simulink model "suspend_kamotu_kato"  (R2020b)
settings: Solver=ode45  StartTime=0.0  StopTime=100
undefined symbols (not defined in the file or in its folder): traj
settings Model: Creator=iketa  LastModifiedBy=kt012
settings DebuggingCC: ArithmeticOperatorsInVariantConditions=warning
settings SFSimCC: CustomCodeUndefinedFunction=UseInterfaceOnly

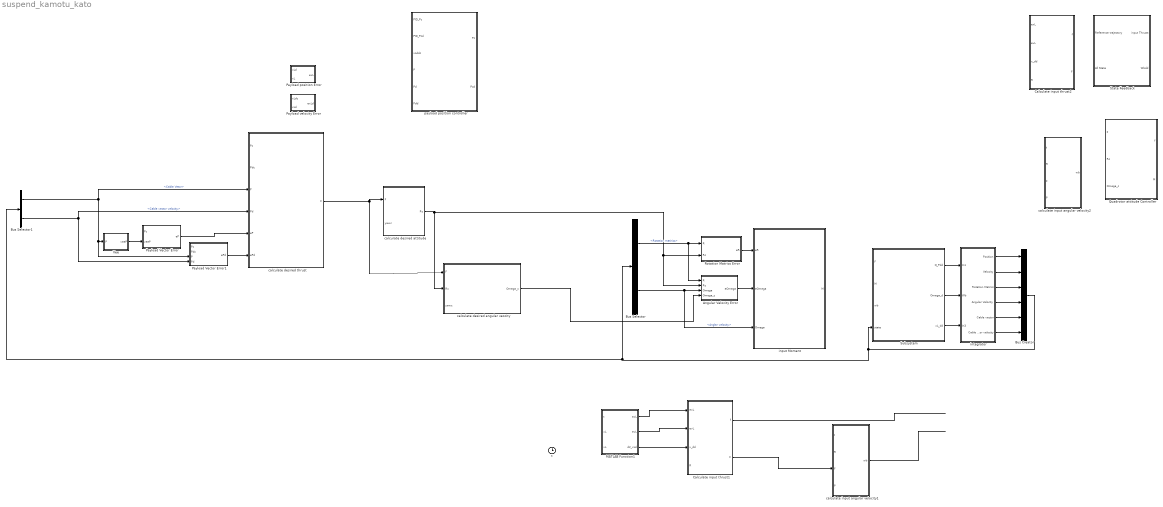
== system suspend_kamotu_kato ==
  Angular Velocity Error : MATLAB Function  TreatAsAtomicUnit=on
  Bus Creator : BusCreator  Inputs=6
  Bus Selector : BusSelector  OutputSignals=Rotation matirics,Anglar velosity
  Bus Selector1 : BusSelector  OutputSignals=Cable Vetor,Cable vector velocity
  Calculate input thrust1 : MATLAB Function
  Calculate input thrust2 : MATLAB Function
  MATLAB Function1 : MATLAB Function  TreatAsAtomicUnit=on
  Payload Vector Error : MATLAB Function  TreatAsAtomicUnit=on
  Payload Vector Error1 : MATLAB Function  TreatAsAtomicUnit=on
  Payload position Error : MATLAB Function  TreatAsAtomicUnit=on
  Payload velocity Error : MATLAB Function  TreatAsAtomicUnit=on
  Quadrotor attitude Controller : MATLAB Function  TreatAsAtomicUnit=on
  Rotation Matrics Error : MATLAB Function  TreatAsAtomicUnit=on
  State Feedback : Subsystem
  Subsystem : Subsystem
  Vee : MATLAB Function  TreatAsAtomicUnit=on
  calculate desired angular veocity : MATLAB Function  TreatAsAtomicUnit=on
  calculate desired thrust : MATLAB Function  TreatAsAtomicUnit=on
  calculate input angular velocity1 : MATLAB Function  TreatAsAtomicUnit=on
  calculate input angular velocity2 : MATLAB Function  TreatAsAtomicUnit=on
  calcurate desired attitude : MATLAB Function  TreatAsAtomicUnit=on
  input Moment : MATLAB Function  TreatAsAtomicUnit=on
  integrator : Subsystem
  payload position controller : MATLAB Function  TreatAsAtomicUnit=on
  t : Clock
  wires:
  Subsystem/1(Q_Pdd) -> integrator/1(In1)
  Subsystem/2(Omega_d) -> integrator/2(Wb)
  Subsystem/3(xL_dd) -> integrator/3(In3)
  ? -> Calculate input thrust1/4(R), calculate input angular velocity1/2(R)
  ? -> MATLAB Function1/3(vL)
  ? -> MATLAB Function1/2(xL), calculate input angular velocity1/4(P)
  calculate input angular velocity1/1(wb) -> ?
  Calculate input thrust1/1(f) -> ?
  Calculate input thrust1/2(F) -> calculate input angular velocity1/3(F)
  MATLAB Function1/3(d2_xLd) -> Calculate input thrust1/3(x_dd)
  MATLAB Function1/2(evL) -> Calculate input thrust1/2(evL)
  ? -> calculate input angular velocity1/1(t)
  MATLAB Function1/1(exL) -> Calculate input thrust1/1(exL)
  integrator/1(Position) -> Bus Creator/1
  integrator/6(Cable vector velocity) -> Bus Creator/6
  integrator/2(Velocity) -> Bus Creator/2
  integrator/3(Rotation Matrics) -> Bus Creator/3
  integrator/5(Cable vector) -> Bus Creator/5
  Bus Creator/1 -> Bus Selector1/1, Bus Selector/1, Subsystem/4(state)
  Angular Velocity Error/1(eOmega) -> input Moment/2(eOmega)
  Rotation Matrics Error/1(eR) -> input Moment/1(eR)
  integrator/4(Angular Velocity) -> Bus Creator/4
  Bus Selector/2 -> input Moment/3(Omega), Angular Velocity Error/3(Omega)  "<Anglar velosity>"
  Bus Selector/1 -> Angular Velocity Error/1(R), Rotation Matrics Error/1(R)  "<Rotation matirics>"
  Vee/1(veeP) -> Payload Vector Error/2(veeP)
  Payload Vector Error/1(eP) -> calculate desired thrust/5(eP)
  Payload Vector Error1/1(ePd) -> calculate desired thrust/6(ePd)
  calculate desired thrust/1(F) -> calcurate desired attitude/1(F), calculate desired angular veocity/1(F)
  calcurate desired attitude/1(Rc) -> Angular Velocity Error/2(Rc), Rotation Matrics Error/2(Rc), calculate desired angular veocity/2(Rc)
  Bus Selector1/1 -> calculate desired thrust/3(P), Payload Vector Error1/3(P), Vee/1(P)  "<Cable Vetor>"
  Bus Selector1/2 -> Payload Vector Error1/4(Pd), calculate desired thrust/4(Pd)  "<Cable vector velocity>"
  calculate desired angular veocity/1(Omega_c) -> Angular Velocity Error/4(Omega_c)

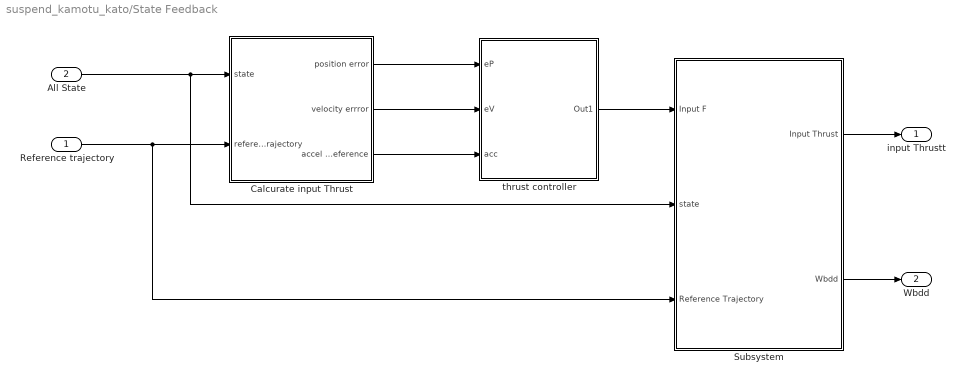
== system suspend_kamotu_kato/State Feedback ==
  Reference trajectory : Inport
  All State : Inport  Port=2
  Calcurate input Thrust : Subsystem
  Subsystem : Subsystem
  thrust controller : Subsystem
  input Thrustt : Outport
  "Wbdd " : Outport  Port=2  VectorParamsAs1DForOutWhenUnconnected=off
  wires:
  thrust controller/1(Out1) -> Subsystem/1(Input F)
  Calcurate input Thrust/3(accel reference) -> thrust controller/3(acc)
  Calcurate input Thrust/2(velocity errror) -> thrust controller/2(eV)
  Calcurate input Thrust/1(position error) -> thrust controller/1(eP)
  Subsystem/1(Input Thrust) -> input Thrustt/1
  Subsystem/2("Wbdd ") -> "Wbdd "/1
  Reference trajectory/1 -> Subsystem/3(Reference Trajectory), Calcurate input Thrust/2(reference trajectory)
  All State/1 -> Subsystem/2(state), Calcurate input Thrust/1(state)

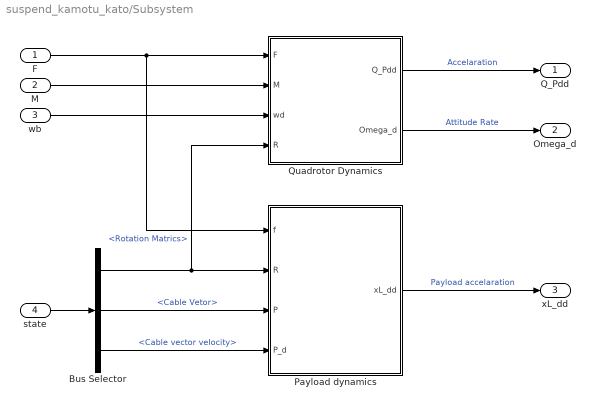
== system suspend_kamotu_kato/Subsystem ==
  F : Inport
  M : Inport  Port=2
  wb : Inport  Port=3
  state : Inport  Port=4
  Bus Selector : BusSelector  OutputSignals=Rotation Matrics,Cable Vetor,Cable vector velocity
  Payload dynamics : MATLAB Function  TreatAsAtomicUnit=on
  Quadrotor Dynamics : MATLAB Function  TreatAsAtomicUnit=on
  Q_Pdd : Outport
  Omega_d : Outport  Port=2
  xL_dd : Outport  Port=3
  wires:
  Payload dynamics/1(xL_dd) -> xL_dd/1  "Payload accelaration"
  Bus Selector/2 -> Payload dynamics/3(P)  "<Cable Vetor>"
  F/1 -> Payload dynamics/1(f), Quadrotor Dynamics/1(F)
  Quadrotor Dynamics/2(Omega_d) -> Omega_d/1  "Attitude Rate"
  Quadrotor Dynamics/1(Q_Pdd) -> Q_Pdd/1  "Accelaration"
  wb/1 -> Quadrotor Dynamics/3(wd)
  state/1 -> Bus Selector/1
  Bus Selector/1 -> Quadrotor Dynamics/4(R), Payload dynamics/2(R)  "<Rotation Matrics>"
  Bus Selector/3 -> Payload dynamics/4(P_d)  "<Cable vector velocity>"
  M/1 -> Quadrotor Dynamics/2(M)

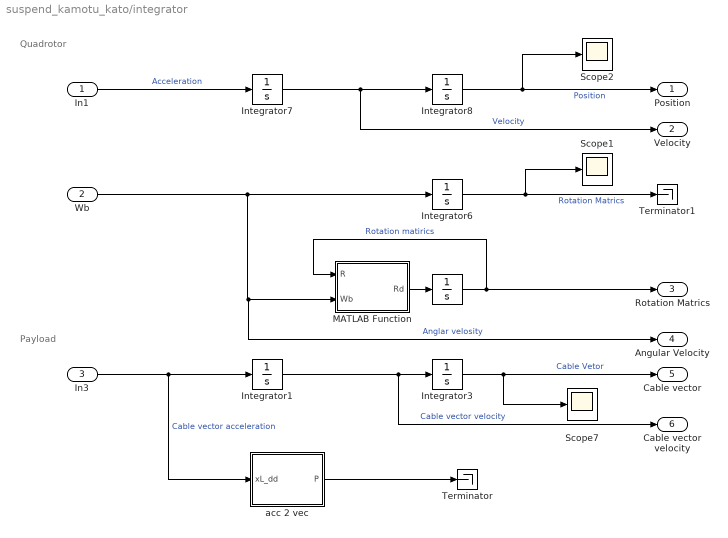
== system suspend_kamotu_kato/integrator ==
  note: Quadrotor
  note: Payload
  In1 : Inport
  Wb : Inport  Port=2
  In3 : Inport  Port=3
  " " : Integrator  InitialCondition=[1 0 0; 0 1 0; 0 0 1];  ContinuousStateAttributes="\"\""
  Integrator{1,3,6..8} (5 alike) : Integrator  InitialCondition=[0;0;0]
  MATLAB Function : MATLAB Function  TreatAsAtomicUnit=on
  Scope1 : Scope
  Scope2 : Scope
  Scope7 : Scope
  Terminator : Terminator
  Terminator1 : Terminator
  acc 2 vec : MATLAB Function  TreatAsAtomicUnit=on
  Position : Outport
  Velocity : Outport  Port=2
  Rotation Matrics : Outport  Port=3
  Angular Velocity : Outport  Port=4
  Cable vector : Outport  Port=5
  Cable vector velocity : Outport  Port=6
  wires:
  In3/1 -> Integrator1/1, acc 2 vec/1(xL_dd)  "Cable vector acceleration"
  Integrator1/1 -> Cable vector velocity/1, Integrator3/1  "Cable vector velocity"
  acc 2 vec/1(P) -> Terminator/1
  Integrator3/1 -> Cable vector/1, Scope7/1  "Cable Vetor"
  Integrator6/1 -> Terminator1/1, Scope1/1  "Rotation Matrics"
  Integrator7/1 -> Velocity/1, Integrator8/1  "Velocity"
  Integrator8/1 -> Position/1, Scope2/1  "Position"
  In1/1 -> Integrator7/1  "Acceleration"
  MATLAB Function/1(Rd) -> " "/1
  Wb/1 -> Angular Velocity/1, MATLAB Function/2(Wb), Integrator6/1  "Anglar velosity"
  " "/1 -> Rotation Matrics/1, MATLAB Function/1(R)  "Rotation matirics"

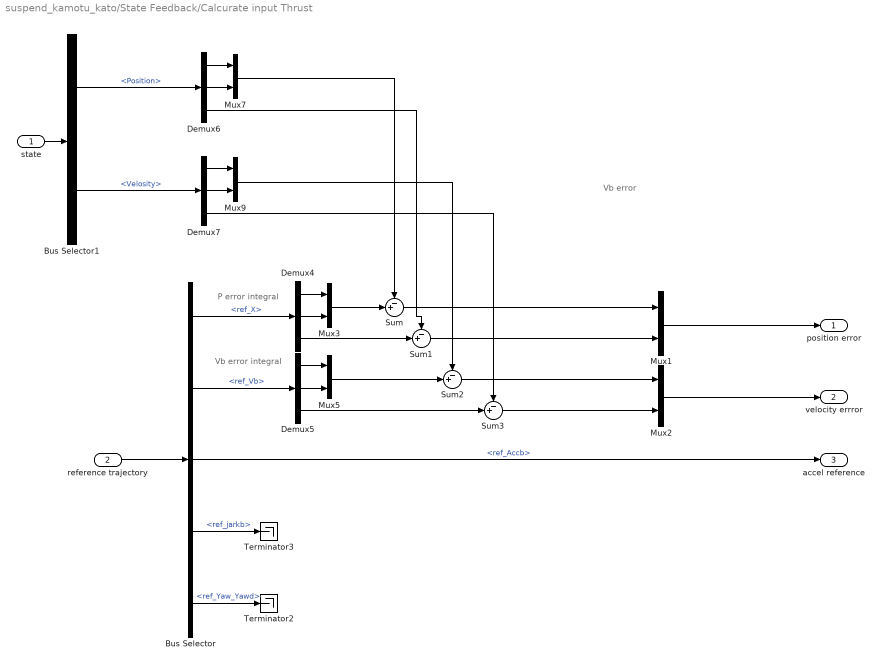
== system suspend_kamotu_kato/State Feedback/Calcurate input Thrust ==
  note: Vb error integral
  note: Vb error
  note: P error integral
  state : Inport
  reference trajectory : Inport  Port=2
  Bus Selector : BusSelector  OutputSignals=ref_X,ref_Vb,ref_Accb,ref_jarkb,ref_Yaw_Yawd
  Bus Selector1 : BusSelector  OutputSignals=Position,Velosity
  Demux{4..7} (4 alike) : Demux  Outputs=3
  Mux{1..3,5,7,9} (6 alike) : Mux  Inputs=2
  Sum{,1..3} (4 alike) : Sum  Inputs=-+|
  Terminator2 : Terminator
  Terminator3 : Terminator
  position error : Outport
  velocity errror : Outport  Port=2
  accel reference : Outport  Port=3
  wires:
  Mux3/1 -> Sum/2
  Demux5/1 -> Mux5/1
  Demux6/3 -> Sum1/1
  Demux7/2 -> Mux9/2
  Bus Selector/2 -> Demux5/1  "<ref_Vb>"
  Demux7/1 -> Mux9/1
  Sum/1 -> Mux1/1
  Demux5/2 -> Mux5/2
  Demux4/2 -> Mux3/2
  Bus Selector1/2 -> Demux7/1  "<Velosity>"
  Sum1/1 -> Mux1/2
  Mux9/1 -> Sum2/1
  Mux7/1 -> Sum/1
  Mux1/1 -> position error/1
  Demux7/3 -> Sum3/1
  Demux6/1 -> Mux7/1
  Bus Selector1/1 -> Demux6/1  "<Position>"
  Sum2/1 -> Mux2/1
  Demux4/3 -> Sum1/2
  state/1 -> Bus Selector1/1
  Bus Selector/3 -> accel reference/1  "<ref_Accb>"
  Demux4/1 -> Mux3/1
  Mux2/1 -> velocity errror/1
  Bus Selector/4 -> Terminator3/1  "<ref_jarkb>"
  Sum3/1 -> Mux2/2
  Bus Selector/5 -> Terminator2/1  "<ref_Yaw_Yawd>"
  Mux5/1 -> Sum2/2
  reference trajectory/1 -> Bus Selector/1
  Bus Selector/1 -> Demux4/1  "<ref_X>"
  Demux5/3 -> Sum3/2
  Demux6/2 -> Mux7/2

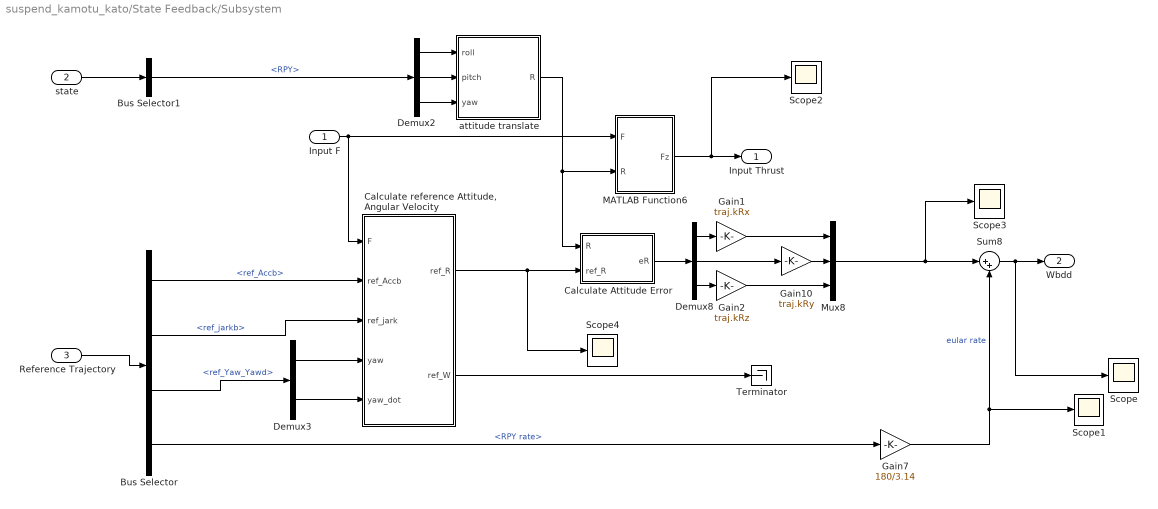
== system suspend_kamotu_kato/State Feedback/Subsystem ==
  Input F : Inport
  state : Inport  Port=2
  Reference Trajectory : Inport  Port=3
  Bus Selector : BusSelector  OutputSignals=ref_Accb,ref_jarkb,ref_Yaw_Yawd,RPY rate
  Bus Selector1 : BusSelector  OutputSignals=RPY
  Calculate Attitude Error : MATLAB Function  TreatAsAtomicUnit=on
  "Calculate reference Attitude, Angular Velocity" : MATLAB Function  TreatAsAtomicUnit=on
  Demux2 : Demux  Outputs=3
  Demux3 : Demux  Outputs=2
  Demux8 : Demux  Outputs=3
  Gain1 : Gain  Gain=traj.kRx
  Gain10 : Gain  Gain=traj.kRy
  Gain2 : Gain  Gain=traj.kRz
  Gain7 : Gain  Gain=180/3.14
  MATLAB Function6 : MATLAB Function
  Mux8 : Mux  Inputs=3
  Scope{,1..4} (5 alike) : Scope
  Sum8 : Sum  Inputs=|++
  Terminator : Terminator
  attitude translate : MATLAB Function  TreatAsAtomicUnit=on
  Input Thrust : Outport
  "Wbdd " : Outport  Port=2  VectorParamsAs1DForOutWhenUnconnected=off
  wires:
  Gain7/1 -> Scope1/1, Sum8/2  "eular rate"
  Gain2/1 -> Mux8/3
  Gain1/1 -> Mux8/1
  Mux8/1 -> Sum8/1, Scope3/1
  Bus Selector/4 -> Gain7/1  "<RPY rate>"
  "Calculate reference Attitude, Angular Velocity"/2(ref_W) -> Terminator/1
  Calculate Attitude Error/1(eR) -> Demux8/1
  Demux2/3 -> attitude translate/3(yaw)
  Demux2/2 -> attitude translate/2(pitch)
  Demux2/1 -> attitude translate/1(roll)
  Bus Selector/2 -> "Calculate reference Attitude, Angular Velocity"/3(ref_jark)  "<ref_jarkb>"
  MATLAB Function6/1(Fz) -> Input Thrust/1, Scope2/1
  state/1 -> Bus Selector1/1
  Demux3/2 -> "Calculate reference Attitude, Angular Velocity"/5(yaw_dot)
  Demux3/1 -> "Calculate reference Attitude, Angular Velocity"/4(yaw)
  Bus Selector/1 -> "Calculate reference Attitude, Angular Velocity"/2(ref_Accb)  "<ref_Accb>"
  Reference Trajectory/1 -> Bus Selector/1
  Bus Selector/3 -> Demux3/1  "<ref_Yaw_Yawd>"
  Bus Selector1/1 -> Demux2/1  "<RPY>"
  Gain10/1 -> Mux8/2
  Demux8/1 -> Gain1/1
  attitude translate/1(R) -> MATLAB Function6/2(R), Calculate Attitude Error/1(R)
  Demux8/2 -> Gain10/1
  Input F/1 -> MATLAB Function6/1(F), "Calculate reference Attitude, Angular Velocity"/1(F)
  Sum8/1 -> "Wbdd "/1, Scope/1
  "Calculate reference Attitude, Angular Velocity"/1(ref_R) -> Calculate Attitude Error/2(ref_R), Scope4/1
  Demux8/3 -> Gain2/1

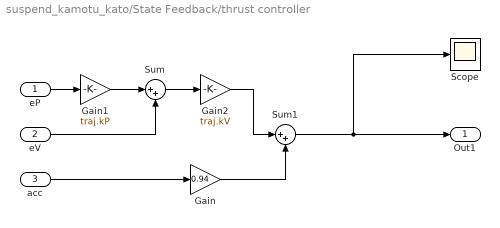
== system suspend_kamotu_kato/State Feedback/thrust controller ==
  eP : Inport
  eV : Inport  Port=2
  acc : Inport  Port=3
  Gain : Gain  Gain=0.94
  Gain1 : Gain  Gain=traj.kP
  Gain2 : Gain  Gain=traj.kV
  Scope : Scope
  Sum : Sum  Inputs=|++
  Sum1 : Sum  Inputs=|++
  Out1 : Outport
  wires:
  Gain/1 -> Sum1/2
  Gain2/1 -> Sum1/1
  Gain1/1 -> Sum/1
  eV/1 -> Sum/2
  eP/1 -> Gain1/1
  Sum1/1 -> Out1/1, Scope/1
  Sum/1 -> Gain2/1
  acc/1 -> Gain/1

== matlab function suspend_kamotu_kato/State Feedback/Subsystem/Calculate reference Attitude, Angular Velocity ==
  data: ref_R output; ref_W output; F input; ref_Accb input; ref_jark input; yaw input; yaw_dot input
function [ref_R, ref_W]= fcn(F, ref_Accb, ref_jark, yaw, yaw_dot)

% Flat Outputから内部状態と入力揚力を計算

m = 0.027;
% 各軸の単位行列
e1 = [1; 0; 0];e2 = [0; 1; 0];e3 = [0; 0; 1];
% ドローンの質量　重力加速度
mQ = 1; g = 9.8;

Xc = [cos(yaw) sin(yaw) 0]';          % よー角のベクトル　Rc(3)
Yc = [-sin(yaw) cos(yaw) 0]';
dXc = yaw_dot * Yc; % よー角のベクトルの微分
dYc = -yaw_dot * Xc; 
   
% 所望の姿勢を計算している
% 軌道の加速度のベクトル: b3 を計算
Zb = F / norm(F);   
%
Xb = cross(Yc, Zb)/norm(cross(Yc, Zb));
Yb = cross(Zb, Xb);
ref_R = [Xb Yb Zb] ;

% 加加速度ベクトルを計算
dfZb = ref_jark;
  
% 目標の姿勢のz軸方向のベクトルの微分を計算
dZb = dfZb/norm(F) - F * dot(F, dfZb)/norm(F)^3; % Zb_dot---------- dot(　fb1/norm(fb1) )

% 目標の姿勢のx軸方向のベクトルを計算
dnorm_Zb_Xc2 = norm(cross(dYc, Zb) + cross(Yc, dZb));
dXb = (cross(dYc, Zb) + cross(Yc, dZb))/dnorm_Zb_Xc2 - cross(Yc, Zb) * dot(cross(Yc, Zb),( cross(dYc, Zb) + cross(Yc, dZb)))/dnorm_Zb_Xc2^3;
   
% 目標の姿勢のy軸方向のベクトルを計算
dYb = cross(dZb, Xb) + cross(Zb, dXb) ;  %dot_b2 = dotb3とb1 の外積と　b3とdot_b1の外積　の和　--------- dot(cross(b3, b1))


wy = dot(Xb, ref_jark) / dot(Zb, ref_Accb);
wx = - dot(Yb, ref_jark) / dot(Zb, ref_Accb);
wz = (yaw_dot * dot(Xc, Xb) + wy * dot(Yc, Zb))/norm(cross(Yc, Zb));
ref_W = [wx wy wz];

== matlab function suspend_kamotu_kato/Quadrotor attitude Controller ==
  data: F input; f output; Rc input; Omega_c input; M output
function [f,M] = fcn(F, Rc, Omega_c)

F = 0;
M = 0;

== matlab function suspend_kamotu_kato/Rotation Matrics Error ==
  data: R input; eR output; Rc input
function eR = fcn(R, Rc)

eR = (Rc'*R - R'*Rc)/2;

== matlab function suspend_kamotu_kato/Angular Velocity Error ==
  data: R input; eOmega output; Rc input; Omega input; Omega_c input
function eOmega = fcn(R, Rc, Omega, Omega_c)

eOmega = Omega - R'*Rc*Omega_c;

== matlab function suspend_kamotu_kato/State Feedback/Subsystem/MATLAB Function6 ==
  data: F input; Fz output; R input
function Fz = fcn(F, R)
e3 = [0;0;1];
u = dot(F, R*e3);

Fz = u;

== matlab function suspend_kamotu_kato/State Feedback/Subsystem/attitude translate ==
  data: roll input; R output; pitch input; yaw input
function R = fcn(roll, pitch, yaw)
% RPYから回転行列計算

R3 = [ cos(yaw) -sin(yaw) 0; sin(yaw) cos(yaw) 0; 0 0 1];              % ヨー角
R2 = [ cos(pitch) 0 sin(pitch); 0 1 0; -sin(pitch) 0 cos(pitch) ];     % ピッチ角
R1 = [ 1 0 0; 0 cos(roll) -sin(roll); 0 sin(roll) cos(roll)];          % ロール角

R = R3* R2 * R1;   % 回転行列（ボディー　-> ワールド）3

== matlab function suspend_kamotu_kato/input Moment ==
  data: eR input; eOmega input; M output; Omega input
function M = fcn(eR, eOmega, Omega)

p = paramdef;
M = -p.kR*eR - p.kOmega*eOmega + cross(Omega, p.I*Omega); %- p.I*(cross(Omegavee, R'*Rc*Omega_c) - R'*Rc*Omega_d);

== matlab function suspend_kamotu_kato/integrator/acc 2 vec ==
  data: xL_dd input; P output
function P  = fcn(xL_dd)                 
g = 9.8;
P = -(xL_dd + g * [0;0;1])/norm(xL_dd + g * [0;0;1]);%ケーブルベクトル

== matlab function suspend_kamotu_kato/integrator/MATLAB Function ==
  data: R input; Rd output; Wb input
function Rd = fcn(R, Wb)
wx = Wb(1);
wy = Wb(2);
wz = Wb(3);
Wb = [ 0    -wz   wy;
       wz    0   -wx;
      -wy    wx   0];
Rd = R * Wb;

== matlab function suspend_kamotu_kato/Payload Vector Error ==
  data: Pc input; veeP input; eP output
function eP = fcn(Pc, veeP)

eP = veeP^2 * Pc:

== matlab function suspend_kamotu_kato/Calculate input thrust1 ==
  data: exL input; f output; evL input; x_dd input; R input; F output
function [f, F]= fcn(exL,evL,x_dd,R)
e3 = [0;0;1];
p = paramdef;

kx_x = 0.2;
kx_y = 0.2;
kx_z = 0.5;

kv_x = 15;
kv_y = 15;
kv_z = 50;

ex_x = kx_x*exL(1);
ex_y = kx_y*exL(2);
ex_z = kx_z*exL(3);
ex_d = [ex_x; ex_y; ex_z];

ev_x = kv_x*evL(1);
ev_y = kv_y*evL(2);
ev_z = kv_z*evL(3);
ev_d = [ev_x; ev_y; ev_z];
 
u = dot(-ex_d - ev_d + p.mQ*x_dd, R*e3);
F = -ex_d - ev_d + mQ*x_dd;

f = u;

== matlab function suspend_kamotu_kato/Vee ==
  data: P input; veeP output
function veeP= fcn(P)
veeP = [0 -P(3) P(2); P(3) 0 -P(1); -P(2) P(1) 0];

== matlab function suspend_kamotu_kato/Payload Vector Error1 ==
  data: Pc input; Pdc input; P input; ePd output; Pd input
function ePd = fcn(Pc,Pdc, P, Pd)

ePd = Pd - cross(cross(Pc, Pdc), P);

== matlab function suspend_kamotu_kato/calculate desired thrust ==
  data: Pc input; Pdc input; P input; F output; Pd input; eP input; ePd input
function F = fcn( Pc, Pdc, P, Pd, eP, ePd)

p = paramdef;
% ----- input thrust calculation ----
F = p.mQ*p.L * (-p.kp*eP - p.kpd*ePd + dot(P, cross(Pc, Pdc))*cross(P, Pd)...
    )-dot(Pc, P)*Pc ;%+ p.mQ*p.L *cross(cross(Pc, Pddc), P);

== matlab function suspend_kamotu_kato/calcurate desired attitude ==
  data: F input; Rc output; yawc input
function Rc = fcn(F, yawc)

b3c = norm(F);
c1c = [cos(yawc); sin(yawc); 0];
c2c = [-sin(yawc) cos(yawc) 0]';

b1c = cross(cross(b3c, c1c)/norm(cross(b3c, c1c)), b3c);
b2c = cross(b3c, c1c)/norm(cross(b3c, c1c));
Rc = [b1c; b2c; b3c];

== matlab function suspend_kamotu_kato/calculate desired angular veocity ==
  data: F input; Omega_c output; Rc input; yawc input
function Omega_c = fcn(F, Rc, yawc)

b1c = zeros(3, 1);b2c = zeros(3, 1);b3c = zeros(3, 1);

b1c = Rc(:, 1);
b2c = Rc(:, 2);

b3c = F/norm(F);
c1c = [cos(yawc); sin(yawc); 0];
c2c = [-sin(yawc) cos(yawc) 0]';

wy = dot(b1c, jarkc) / dot(b3c, F);
wx = - dot(b2c, jarkc) / dot(b3c, F);
wz = (yawdc * dot(c1c, b1c) + wy * dot(c2c, b3c))/norm(cross(c2c, b3c));
ref_W = [wx wy wz];
Omega_c = [0,-wz,wy; wz,0,-wx; -wy,wx,0];

== matlab function suspend_kamotu_kato/Payload position Error ==
  data: xLd input; exL output; xL input
function exL = fcn(xLd, xL)

exL = xL - xLd;

== matlab function suspend_kamotu_kato/Payload velocity Error ==
  data: xLdc input; exLd output; xLd input
function exLd = fcn(xLdc, xLd)

exLd = xLd - xLdc;

== matlab function suspend_kamotu_kato/payload position controller ==
  data: PID_Pc input; Pc output; PID_Pcd input; xLddc input; P input; Pd input; Pdd input; Pcd output
function [Pc,Pcd] = fcn(PID_Pc, PID_Pcd, xLddc, P, Pd, Pdd)
p = paramdef;
A = (p.mQ + p.mL)*PID_Pc ...
    + (p.mQ + p.mL)*(xLddc + p.g*p.e3) + p.mQ*p.L*dot(Pd, Pd) * P;
Pc = A/norm(A);

Pcd = (p.mQ + p.mL)*PID_Pcd * (p.mQ + p.mL)*(xLddd)...
     + p.mQ*p.L*dot(Pd, Pd) * Pd;% + 2*p.mQ*p.L*dot(Pdd, Pd) * P;

== matlab function suspend_kamotu_kato/Subsystem/Quadrotor Dynamics ==
  data: F input; M input; wd input; Q_Pdd output; R input; Omega_d output
function [Q_Pdd,Omega_d] = fcn(F, M, wd, R)
p = paramdef;
Q_Pdd = (F*R*p.e3/p.mQ) - p.g*p.e3;
Omega_d = pinv(p.I)*(M - cross(wd, p.I*wd));

== matlab function suspend_kamotu_kato/MATLAB Function1 ==
  data: exL output; evL output; t input; xL input; vL input; d2_xLd output
function [exL,evL,d2_xLd] = fcn(t,xL,vL)                 
p = paramdef;
w = 2 * pi/p.T;          % 角周波数

% 中心　半径　　
c = [0;0;0];

xLd = c + p.r*[sin(w*t); cos(w*t); 0];         % 位置の軌道の位置
d_xLd = p.r*[w*cos(w*t); -w*sin(w*t); 0];       % 速度の軌道
d2_xLd = p.r*[-w^2*sin(w*t); -w^2*cos(w*t); 0]; % 加速度の軌道

exL = xL - xLd;
evL = vL - d_xLd;

== matlab function suspend_kamotu_kato/calculate input angular velocity1 ==
  data: t input; wb output; R input; F input; P input
function wb= fcn(t,R, F,P)
p = paramdef;
% 軌道生成
w = 2 * pi/p.T;          % 角周波数

% 中心　半径　　
c = [0;0;0];

% Flat Outputから内部状態と入力揚力を計算
% 各軸の単位行列
e1 = [1; 0; 0];e2 = [0; 1; 0];e3 = [0; 0; 1];
% 重力加速度
g = 9.8;


x = c + p.r*[sin(w*t); cos(w*t); 0] + p.L*P;         % 位置の軌道の位置
dx = p.r*[w*cos(w*t); -w*sin(w*t); 0];       % 速度の軌道
d2x = p.r*[-w^2*sin(w*t); -w^2*cos(w*t); 0]; % 加速度の軌道
d3x = p.r*[-w^3*cos(w*t); w^3*sin(w*t); 0];  % 加加速度の軌道
d4x = p.r*[w^4*sin(w*t); w^4*cos(w*t); 0];   % 加加加速度の軌道

alpha = 0;                                 % よー角の軌道
alpha_dot = 0;                             % よー角速度の軌道
Xc = [cos(alpha) sin(alpha) 0]';          % よー角のベクトル　Rc(3)
Yc = [-sin(alpha) cos(alpha) 0]';
dXc = alpha_dot * Yc; % よー角のベクトルの微分
dYc = -alpha_dot * Xc; 

% 速度，加速度，加加速度の代入
axQ = d2x; 
daxQ = d3x;
d2aQ = d4x;
   
% 所望の姿勢を計算している
% 軌道の加速度のベクトル: b3 を計算
fZb = F;           
norm_fZb = norm(F) ;
Zb = fZb / norm_fZb ;

% 所望の加速度のベクトルと所望のヨー角のベクトル
Zb_Xc = cross(Zb, Xc) ;
   
% オリジナル
Xb = cross(Yc, Zb)/norm(cross(Yc, Zb));
Yb = cross(Zb, Xb);
Rd = [Xb Yb Zb] ;
 
% 加加速度ベクトルを計算
dfZb = p.mQ*(daxQ);
  
% 目標の姿勢のz軸方向のベクトルの微分を計算
dZb = dfZb/norm(fZb) - fZb * dot(fZb, dfZb)/norm(fZb)^3; % Zb_dot---------- dot(　fb1/norm(fb1) )

% 目標の姿勢のx軸方向のベクトルを計算
dnorm_Zb_Xc2 = norm(cross(dYc, Zb) + cross(Yc, dZb));
dXb = (cross(dYc, Zb) + cross(Yc, dZb))/dnorm_Zb_Xc2 - cross(Yc, Zb) * dot(cross(Yc, Zb),( cross(dYc, Zb) + cross(Yc, dZb)))/dnorm_Zb_Xc2^3;
   
% 目標の姿勢のy軸方向のベクトルを計算
dYb = cross(dZb, Xb) + cross(Zb, dXb) ;  %dot_b2 = dotb3とb1 の外積と　b3とdot_b1の外積　の和　--------- dot(cross(b3, b1))

R_T = R';
Rd_T = Rd';
eR = (Rd_T*R - R_T*Rd)/2;

wy = dot(Xb, daxQ) / dot(Zb, F); 
wx = - dot(Yb, daxQ) / dot(Zb, F); 
wz = (alpha_dot * dot(Xc, Xb) + wy * dot(Yc, Zb))/norm(cross(Yc, Zb));
wd = [0 -wz wy;wz 0 -wx; -wy wx 0];


kR = 1.0;

u = -kR * eR + wd;

wb = u;

== matlab function suspend_kamotu_kato/calculate input angular velocity2 ==
  data: t input; wb output; R input; F input; P input
function wb= fcn(t,R, F,P)
p = paramdef;
% 軌道生成
w = 2 * pi/p.T;          % 角周波数

% 中心　半径　　
c = [0;0;0];

% Flat Outputから内部状態と入力揚力を計算
% 各軸の単位行列
e1 = [1; 0; 0];e2 = [0; 1; 0];e3 = [0; 0; 1];
% 重力加速度
g = 9.8;


x = c + p.r*[sin(w*t); cos(w*t); 0] + p.L*P;         % 位置の軌道の位置
dx = p.r*[w*cos(w*t); -w*sin(w*t); 0];       % 速度の軌道
d2x = p.r*[-w^2*sin(w*t); -w^2*cos(w*t); 0]; % 加速度の軌道
d3x = p.r*[-w^3*cos(w*t); w^3*sin(w*t); 0];  % 加加速度の軌道
d4x = p.r*[w^4*sin(w*t); w^4*cos(w*t); 0];   % 加加加速度の軌道

alpha = 0;                                 % よー角の軌道
alpha_dot = 0;                             % よー角速度の軌道
Xc = [cos(alpha) sin(alpha) 0]';          % よー角のベクトル　Rc(3)
Yc = [-sin(alpha) cos(alpha) 0]';
dXc = alpha_dot * Yc; % よー角のベクトルの微分
dYc = -alpha_dot * Xc; 

% 速度，加速度，加加速度の代入
axQ = d2x; 
daxQ = d3x;
d2aQ = d4x;
   
% 所望の姿勢を計算している
% 軌道の加速度のベクトル: b3 を計算
fZb = F;           
norm_fZb = norm(F) ;
Zb = fZb / norm_fZb ;

% 所望の加速度のベクトルと所望のヨー角のベクトル
Zb_Xc = cross(Zb, Xc) ;
   
% オリジナル
Xb = cross(Yc, Zb)/norm(cross(Yc, Zb));
Yb = cross(Zb, Xb);
Rd = [Xb Yb Zb] ;
 
% 加加速度ベクトルを計算
dfZb = p.mQ*(daxQ);
  
% 目標の姿勢のz軸方向のベクトルの微分を計算
dZb = dfZb/norm(fZb) - fZb * dot(fZb, dfZb)/norm(fZb)^3; % Zb_dot---------- dot(　fb1/norm(fb1) )

% 目標の姿勢のx軸方向のベクトルを計算
dnorm_Zb_Xc2 = norm(cross(dYc, Zb) + cross(Yc, dZb));
dXb = (cross(dYc, Zb) + cross(Yc, dZb))/dnorm_Zb_Xc2 - cross(Yc, Zb) * dot(cross(Yc, Zb),( cross(dYc, Zb) + cross(Yc, dZb)))/dnorm_Zb_Xc2^3;
   
% 目標の姿勢のy軸方向のベクトルを計算
dYb = cross(dZb, Xb) + cross(Zb, dXb) ;  %dot_b2 = dotb3とb1 の外積と　b3とdot_b1の外積　の和　--------- dot(cross(b3, b1))

R_T = R';
Rd_T = Rd';
eR = (Rd_T*R - R_T*Rd)/2;

wy = dot(Xb, daxQ) / dot(Zb, F); 
wx = - dot(Yb, daxQ) / dot(Zb, F); 
wz = (alpha_dot * dot(Xc, Xb) + wy * dot(Yc, Zb))/norm(cross(Yc, Zb));
wd = [0 -wz wy;wz 0 -wx; -wy wx 0];


kR = 1.0;

u = -kR * eR + wd;

wb = u;

== matlab function suspend_kamotu_kato/Subsystem/Payload dynamics ==
  data: f input; R input; P input; xL_dd output; P_d input
function xL_dd  = fcn(f,R,P,P_d)                 
g = 9.8;
e3 = [0;0;1];
p = paramdef;
xL_dd = {(P*f*R*e3 -p.mQ*p.L*(dot(P_d,P_d))*P)/(p.mQ + p.mL)} - g*e3;

== matlab function suspend_kamotu_kato/Calculate input thrust2 ==
  data: exL input; f output; evL input; x_dd input; R input; F output
function [f, F]= fcn(exL,evL,x_dd,R)
e3 = [0;0;1];
p = paramdef;

kx_x = 0.2;
kx_y = 0.2;
kx_z = 0.5;

kv_x = 15;
kv_y = 15;
kv_z = 50;

ex_x = kx_x*exL(1);
ex_y = kx_y*exL(2);
ex_z = kx_z*exL(3);
ex_d = [ex_x; ex_y; ex_z];

ev_x = kv_x*evL(1);
ev_y = kv_y*evL(2);
ev_z = kv_z*evL(3);
ev_d = [ev_x; ev_y; ev_z];
 
u = dot(-ex_d - ev_d + p.mQ*x_dd, R*e3);
F = -ex_d - ev_d + mQ*x_dd;

f = u;

== matlab function suspend_kamotu_kato/State Feedback/Subsystem/Calculate Attitude Error ==
  data: R input; ref_R input; eR output
function eR = fcn(R, ref_R)
transpose_R = R';
transpose_ref_R = ref_R';
tmp = -(transpose_ref_R*R - transpose_R*ref_R)/2;
eR = [tmp(3, 2), -tmp(3, 1), tmp(2, 1)];
